simulink model "Prac_2_Q1_3"  (R2020a)
settings: Solver=VariableStepAuto  StartTime=0.0  StopTime=20  RelTol=1e-3
values from neighbouring files (symbols this model uses):
  inputAmp = 50    [Prac_2.m]
  inputBias = 40    [Prac_2.m]
  rangeMax = 115    [Prac_2.m]
  rangeMin = -15    [Prac_2.m]
  sampleTime = 0.2    [Prac_2.m]
  Sens = 45.9/1000    (= 0.0459)    [Prac_2.m]
libraries: simulink x1, simulink_extras x1, cstblocks x1
settings Model: Creator=kaibr  LastModifiedBy=kaibr

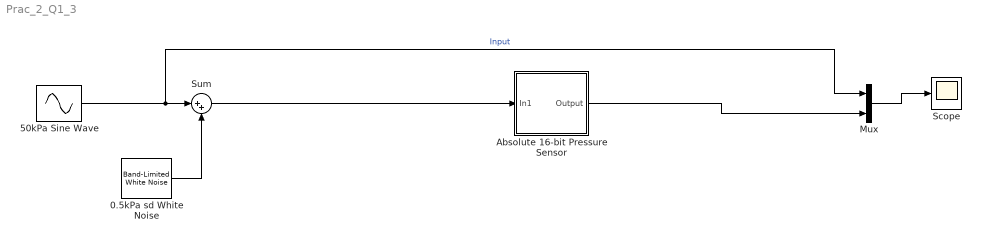
== system Prac_2_Q1_3 ==
  0.5kPa sd White Noise : simulink/Sources/Band-Limited White Noise  Cov=noisePow  Ts=sampleTime  seed=[23341]
  50kPa Sine Wave : Sin  Amplitude=inputAmp  Bias=inputBias  Frequency=0.5  SampleTime=sampleTime
  Absolute 16-bit Pressure Sensor : Subsystem  mask(16-Bit Absolute pressure Sensor){}
      mask help:
      | A sensor that uses a 16-bit ADC with voltage supply of +-5V to measure pressure in kPa. The range of the sensor is -15kPa to 115kPa.
      | ● Range of 115kPa to -15kPa
      | ● Std. deviation noise (0.5 kPa)
      | ● Sensitivity of 45.9 mV/kPa
      | ● Assume a 5V supply voltage and sampling time of 0.02s (50Hz)
      | ● Sensor lag of 0.5s
      mask Help:
      | A sensor that uses a 16-bit ADC with voltage supply of +-5V to measure pressure in kPa. The range of the sensor is -15kPa to 115kPa.
      | ● Range of 115kPa to -15kPa
      | ● Std. deviation noise (0.5 kPa)
      | ● Sensitivity of 45.9 mV/kPa
      | ● Assume a 5V supply voltage and sampling time of 0.02s (50Hz)
      | ● Sensor lag of 0.5s
      mask DialogControl DescTextVar Prompt: %<Input Pressure (kPa)>
      mask DialogControl Control2 Prompt: Input Pressure (kPa)
      mask Display: image('ad5bc0cd-a5ae-459f-85f7-3cca9d814d60.png'); % Use "Edit Image" on toolstrip to change.
  Mux : Mux  Inputs=2
  Scope : Scope
  Sum : Sum  Inputs=|++
  wires:
  Mux/1 -> Scope/1
  0.5kPa sd White Noise/1 -> Sum/2
  50kPa Sine Wave/1 -> Mux/1, Sum/1  "Input"
  Sum/1 -> Absolute 16-bit Pressure Sensor/1(In1)
  Absolute 16-bit Pressure Sensor/1(Output) -> Mux/2

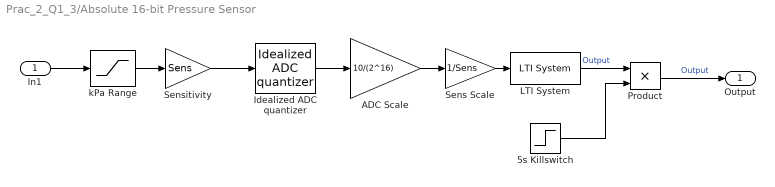
== system Prac_2_Q1_3/Absolute 16-bit Pressure Sensor ==
  In1 : Inport
  5s Killswitch : Step  Time=5  Before=1  After=0  SampleTime=sampleTime
  ADC Scale : Gain  Gain=10/(2^16)
  Idealized ADC quantizer : simulink_extras/Additional Discrete/Idealized ADC quantizer  NumberOfConverterBits=16  Vmin=-5  Vmax=5  OutputDataType=double  OutputNegativeValues=on
  LTI System : cstblocks/LTI System  sys=delayFn  IC=[]
  Product : Product
  Sens Scale : Gain  Gain=1/Sens
  Sensitivity : Gain  Gain=Sens
  kPa Range : Saturate  UpperLimit=rangeMax  LowerLimit=rangeMin
  Output : Outport
  wires:
  kPa Range/1 -> Sensitivity/1
  In1/1 -> kPa Range/1
  Sens Scale/1 -> LTI System/1
  ADC Scale/1 -> Sens Scale/1
  Sensitivity/1 -> Idealized ADC quantizer/1
  Idealized ADC quantizer/1 -> ADC Scale/1
  5s Killswitch/1 -> Product/2
  Product/1 -> Output/1  "Output"
  LTI System/1 -> Product/1  "Output"
